simulink model "OneThrid_block"  (R2022b)
settings: Solver=VariableStepAuto  StartTime=0.0  StopTime=1  RelTol=1e-3
settings Model: Creator=yeyi5  LastModifiedBy=yeyi5

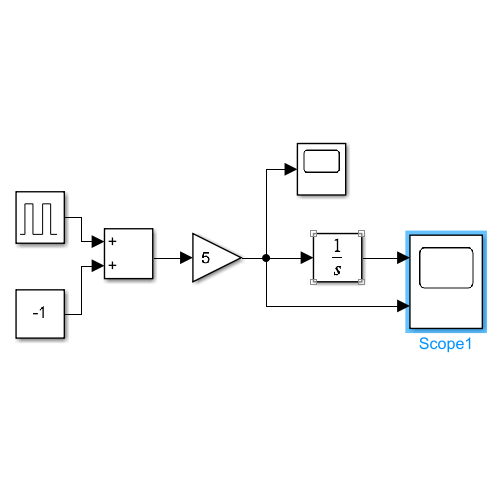
[thumbnail: Simulink's stored preview of the top-level diagram]
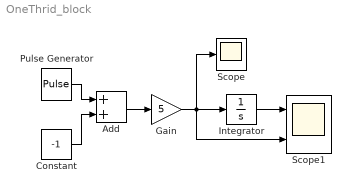
== system OneThrid_block ==
  Add : Sum
  Constant : Constant  Value=-1
  Gain : Gain  Gain=5
  Integrator : Integrator
  Pulse Generator : DiscretePulseGenerator  PulseType=Time based  Amplitude=2  Period=1/5  PulseWidth=50
  Scope : Scope
  Scope1 : Scope  NumInputPorts=2
  wires:
  Pulse Generator/1 -> Add/1
  Constant/1 -> Add/2
  Add/1 -> Gain/1
  Gain/1 -> Scope/1, Scope1/2, Integrator/1
  Integrator/1 -> Scope1/1
